simulink model "ForcePlate"  (R2017b)
settings: Solver=FixedStepDiscrete  StartTime=0.0  StopTime=inf  FixedStep=0.001  RelTol=1e-3  EnableMultiTasking=on
libraries: slrtlib x7, speedgoatlib_IO106 x2
settings Model: sg_rtwmakecfg_data=_sglibc_  Creator=Katie  LastModifiedBy=Vicon-OEM
settings SolverCC: ConcurrentTasks=on  AutoInsertRateTranBlk=on
settings DataIOCC: SaveFormat=StructureWithTime  SaveOutput=off  SaveTime=off
settings OptimizationCC: BlockReduction=off  OptimizeBlockIOStorage=off  BufferReuse=off  GlobalBufferReuse=off  ExpressionFolding=off  LocalBlockOutputs=off
settings HardwareCC: ProdBitPerPointer=32  ProdBitPerSizeT=32  ProdBitPerPtrDiffT=32  ProdLargestAtomicFloat=None  ProdWordSize=32  ProdLongLongMode=on  ProdHWDeviceType=Generic->32-bit x86 compatible
settings RTWCC: SystemTargetFile=slrt.tlc  TemplateMakefile=slrt_default_tmf  Description=Simulink Real-Time  CodeExecutionProfiling=on  RTWCompilerOptimization=on
settings SimulinkRealTimeCC: SupportVariableSizeSignals=on  RL32LogTETModifier=off  xPCConcurrentTasks=on

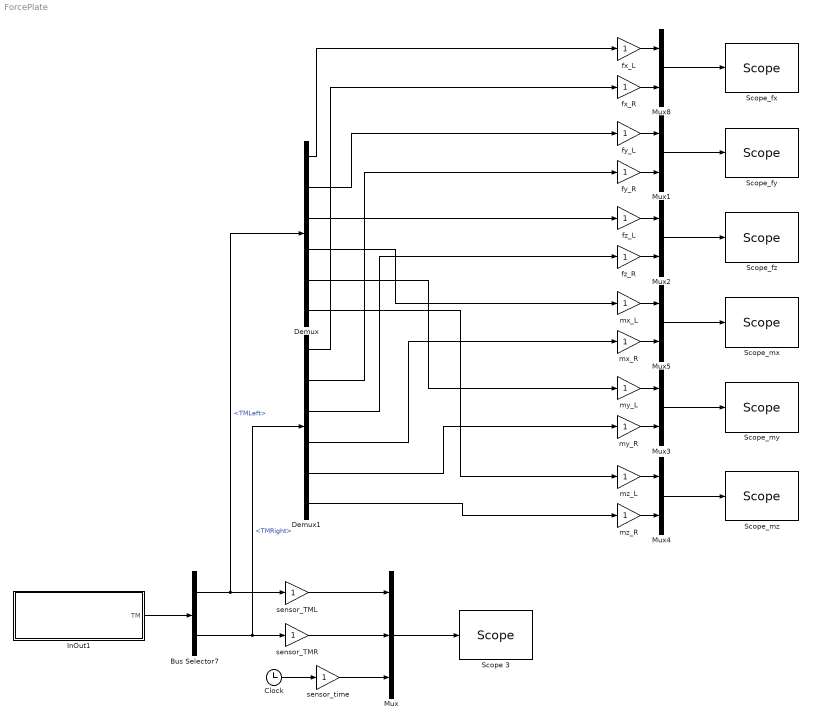
== system ForcePlate ==
  Bus Selector7 : BusSelector  OutputSignals=TMLeft,TMRight
  Clock : Clock
  Demux : Demux  Outputs=6
  Demux1 : Demux  Outputs=6
  InOut1 : Subsystem
  Mux : Mux  Inputs=3
  Mux{1..5,8} (6 alike) : Mux  Inputs=2
  Scope 3 : slrtlib/Displays and Logging/Scope   scopeno=101  scopetype=File  autostart=off  viewmode=Graphical redraw  formatstr='%15.6f'  grid=on  ylimits=[0,0]  nosamples=60*60*1000  noprepostsamples=0  interleave=1  triggermode=FreeRun  triggersignal=1  trigsignalfromport=off  triggerlevel=0.0  triggerslope=Either  triggerscope=1  triggersample=0  filename=pacedTM.dat  mode=Lazy  writesize=512  autorestart=off  dynamicfilemode=off  maxwritefilesize=512*1024^2
  "Scope_fx " : slrtlib/Displays and Logging/Scope   scopeno=1  scopetype=Target  autostart=on  viewmode=Graphical rolling  formatstr='%15.6f'  grid=on  ylimits=[0,0]  nosamples=2*1000/2  noprepostsamples=0  interleave=4  triggermode=FreeRun  triggersignal=1  trigsignalfromport=off  triggerlevel=0.0  triggerslope=Either  triggerscope=1  triggersample=0  filename=data.dat  mode=Lazy  writesize=512  autorestart=off  dynamicfilemode=off  maxwritefilesize=512*1024^2
  Scope_fy : slrtlib/Displays and Logging/Scope   scopeno=2  scopetype=Target  autostart=on  viewmode=Graphical rolling  formatstr='%15.6f'  grid=on  ylimits=[0,0]  nosamples=2*1000/2  noprepostsamples=0  interleave=4  triggermode=FreeRun  triggersignal=1  trigsignalfromport=off  triggerlevel=0.0  triggerslope=Either  triggerscope=1  triggersample=0  filename=data.dat  mode=Lazy  writesize=512  autorestart=off  dynamicfilemode=off  maxwritefilesize=512*1024^2
  Scope_fz : slrtlib/Displays and Logging/Scope   scopeno=3  scopetype=Target  autostart=on  viewmode=Graphical rolling  formatstr='%15.6f'  grid=on  ylimits=[0,0]  nosamples=2*1000/2  noprepostsamples=0  interleave=4  triggermode=FreeRun  triggersignal=1  trigsignalfromport=off  triggerlevel=0.0  triggerslope=Either  triggerscope=1  triggersample=0  filename=data.dat  mode=Lazy  writesize=512  autorestart=off  dynamicfilemode=off  maxwritefilesize=512*1024^2
  Scope_mx : slrtlib/Displays and Logging/Scope   scopeno=4  scopetype=Target  autostart=on  viewmode=Graphical rolling  formatstr='%15.6f'  grid=on  ylimits=[0,0]  nosamples=2*1000/2  noprepostsamples=0  interleave=4  triggermode=FreeRun  triggersignal=1  trigsignalfromport=off  triggerlevel=0.0  triggerslope=Either  triggerscope=1  triggersample=0  filename=data.dat  mode=Lazy  writesize=512  autorestart=off  dynamicfilemode=off  maxwritefilesize=512*1024^2
  Scope_my : slrtlib/Displays and Logging/Scope   scopeno=5  scopetype=Target  autostart=on  viewmode=Graphical rolling  formatstr='%15.6f'  grid=on  ylimits=[0,0]  nosamples=2*1000/2  noprepostsamples=0  interleave=4  triggermode=FreeRun  triggersignal=1  trigsignalfromport=off  triggerlevel=0.0  triggerslope=Either  triggerscope=1  triggersample=0  filename=data.dat  mode=Lazy  writesize=512  autorestart=off  dynamicfilemode=off  maxwritefilesize=512*1024^2
  Scope_mz : slrtlib/Displays and Logging/Scope   scopeno=6  scopetype=Target  autostart=on  viewmode=Graphical rolling  formatstr='%15.6f'  grid=on  ylimits=[0,0]  nosamples=2*1000/2  noprepostsamples=0  interleave=4  triggermode=FreeRun  triggersignal=1  trigsignalfromport=off  triggerlevel=0.0  triggerslope=Either  triggerscope=1  triggersample=0  filename=data.dat  mode=Lazy  writesize=512  autorestart=off  dynamicfilemode=off  maxwritefilesize=512*1024^2
  fx_L : Gain
  fx_R : Gain
  fy_L : Gain
  fy_R : Gain
  fz_L : Gain
  fz_R : Gain
  mx_L : Gain
  mx_R : Gain
  my_L : Gain
  my_R : Gain
  mz_L : Gain
  mz_R : Gain
  sensor_TML : Gain
  sensor_TMR : Gain
  sensor_time : Gain
  wires:
  Mux/1 -> Scope 3/1
  Clock/1 -> sensor_time/1
  InOut1/1(TM) -> Bus Selector7/1
  sensor_TML/1 -> Mux/1
  Bus Selector7/2 -> Demux1/1, sensor_TMR/1  "<TMRight>"
  sensor_TMR/1 -> Mux/2
  sensor_time/1 -> Mux/3
  Bus Selector7/1 -> Demux/1, sensor_TML/1  "<TMLeft>"
  Demux/1 -> fx_L/1
  fx_L/1 -> Mux8/1
  fx_R/1 -> Mux8/2
  Mux8/1 -> "Scope_fx "/1
  Demux1/1 -> fx_R/1
  Mux1/1 -> Scope_fy/1
  fy_L/1 -> Mux1/1
  fy_R/1 -> Mux1/2
  fz_R/1 -> Mux2/2
  fz_L/1 -> Mux2/1
  Mux2/1 -> Scope_fz/1
  Demux/2 -> fy_L/1
  Demux1/2 -> fy_R/1
  Demux/3 -> fz_L/1
  Demux1/3 -> fz_R/1
  Mux5/1 -> Scope_mx/1
  my_R/1 -> Mux3/2
  my_L/1 -> Mux3/1
  Mux3/1 -> Scope_my/1
  mx_R/1 -> Mux5/2
  mz_R/1 -> Mux4/2
  mz_L/1 -> Mux4/1
  mx_L/1 -> Mux5/1
  Mux4/1 -> Scope_mz/1
  Demux/4 -> mx_L/1
  Demux1/4 -> mx_R/1
  Demux/5 -> my_L/1
  Demux1/5 -> my_R/1
  Demux/6 -> mz_L/1
  Demux1/6 -> mz_R/1

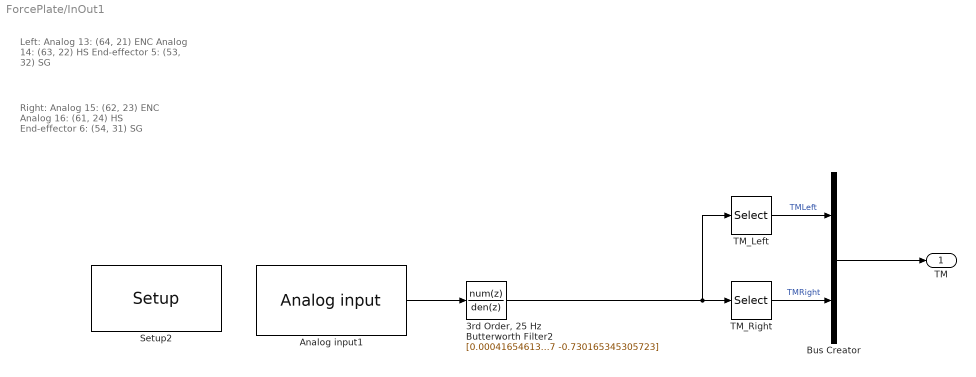
== system ForcePlate/InOut1 ==
  note: Left:
      | Analog 13: (64, 21) ENC
      | Analog 14: (63, 22) HS
      | End-effector 5: (53, 32) SG
  note: Right:
      | Analog 15: (62, 23) ENC
      | Analog 16: (61, 24) HS
      | End-effector 6: (54, 31) SG
  "3rd Order, 25 Hz Butterworth Filter2" : DiscreteFilter  Numerator="[0.000416546139075769\t0.00124963841722731\t0.00124963841722731\t0.000416546139075769]"  Denominator="[1\t-2.68615739654814\t2.41965511096647\t-0.730165345305723]"
  Analog input1 : speedgoatlib_IO106/Analog input  id=1  channels=12  range=1  coupling=1  ts=dt_speedgoat  initiator=1  pciSlot=-1
      settings: SourceProductName=Simulink Real-Time: Speedgoat I/O Driver Library
  Bus Creator : BusCreator  Inputs=2
  Setup2 : speedgoatlib_IO106/Setup  group=Module setup  id=1  cal=on  initiator=Initiator  pciSlot=-1  adChannel=12  adRange=+-10V  adCoupling=Single-ended
      settings: SourceProductName=Simulink Real-Time: Speedgoat I/O Driver Library
  TM_Left : Selector  InputPortWidth=12  IndexOptions=Index vector (dialog)  Indices=1:6  OutputSizes=1
  TM_Right : Selector  InputPortWidth=12  IndexOptions=Index vector (dialog)  Indices=7:12  OutputSizes=1
  TM : Outport
  wires:
  Bus Creator/1 -> TM/1
  Analog input1/1 -> "3rd Order, 25 Hz Butterworth Filter2"/1
  "3rd Order, 25 Hz Butterworth Filter2"/1 -> TM_Right/1, TM_Left/1
  TM_Left/1 -> Bus Creator/1  "TMLeft"
  TM_Right/1 -> Bus Creator/2  "TMRight"
